simulink model "district_heating_r04"  (R2018b)
settings: Solver=ode45  StartTime=0.0  StopTime=24*3600  RelTol=1e-3
undefined symbols (not defined in the file): DPConstant, DPLinear, DPQuadratic, FluidMix, ID, MassFlow, path_carnot, Temperature
libraries: carnot x12, Pipe_BiFlow x2
settings Model: Creator=drhf  LastModifiedBy=drhf
settings SolverCC: AlgebraicLoopSolver=LineSearch

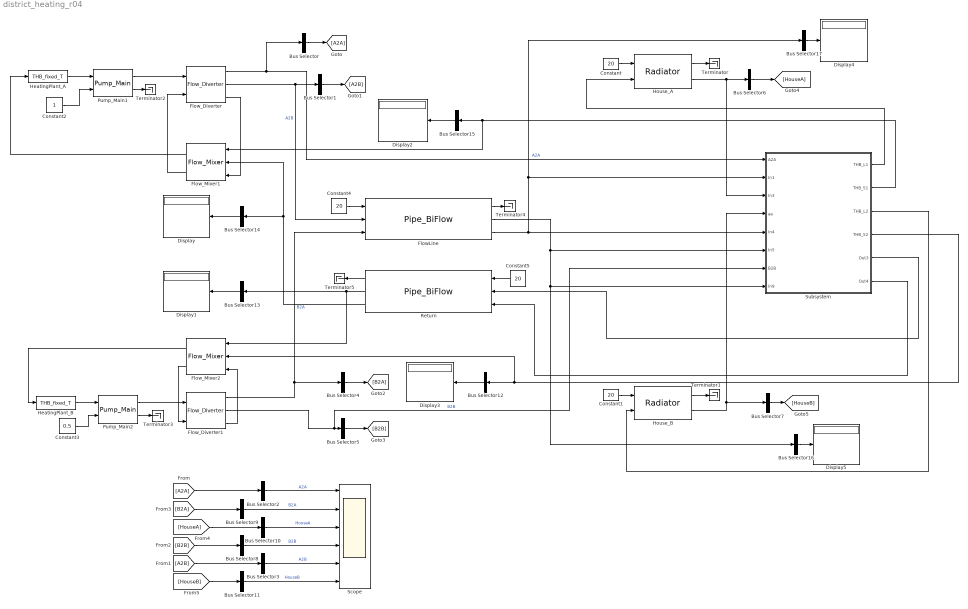
== system district_heating_r04 ==
  Bus Selector{,1,4..7} (6 alike) : BusSelector  OutputSignals=Temperature,MassFlow  OutputAsBus=on
  Bus Selector{2..3,8..11} (6 alike) : BusSelector  OutputSignals=MassFlow  OutputAsBus=on
  Bus Selector{12..17} (6 alike) : BusSelector  OutputSignals=MassFlow,DPConstant,DPLinear,DPQuadratic  OutputAsBus=on
  Constant{,1,4..5} (4 alike) : Constant  Value=20
  Constant2 : Constant
  Constant3 : Constant  Value=0.5
  Display{,1..5} (6 alike) : Display
  FlowLine : Pipe_BiFlow/Pipe_BiFlow  t0=20  hgt=254.6479  stgtype=1  tini=[20 20 20 20 20 20 20 20 20 20]  mpts=[1 2 3 4 5 6 7 8 9 10]  PathName=fullfile(path_carnot('libsl'),'Storage','Thermal','Storage_Type_1','parameter_set')  FileName='<user defined>'  userPath=off  userParam=on  uwall=1  ubot=1  utop=1  axcond=1  volume=2  dia=0.1  standing=standing cylinder  nodes=10  mpoints=10  pipe1inlet=1  pipe1outlet=0  pipe1dia=0.1  pipe2inlet=0  pipe2outlet=1  pipe2dia=0.1
  Flow_Diverter : carnot/Hydraulics/Flow_Diverter
      settings: SourceProductName=Carnot
  Flow_Diverter1 : carnot/Hydraulics/Flow_Diverter
      settings: SourceProductName=Carnot
  Flow_Mixer1 : carnot/Hydraulics/Flow_Mixer
      settings: SourceProductName=Carnot
  Flow_Mixer2 : carnot/Hydraulics/Flow_Mixer
      settings: SourceProductName=Carnot
  HeatingPlant_A : carnot/Source/Simple/THB_fixed_T  t=70
      settings: SourceProductName=Carnot
  HeatingPlant_B : carnot/Source/Simple/THB_fixed_T  t=60
      settings: SourceProductName=Carnot
  House_A : carnot/Source/Heat_Exchanger/Radiator  pnom=500  dtnom=49.83  expo=1.3  mcap=5*4182  tini=20  lin=10  qua=10
      settings: SourceProductName=Carnot
  House_B : carnot/Source/Heat_Exchanger/Radiator  pnom=500  dtnom=49.83  expo=1.3  mcap=5*4182  tini=20  lin=10  qua=10
      settings: SourceProductName=Carnot
  Pump_Main1 : carnot/Hydraulics/Pump_Main  Tini=20  p0=3e5  IDpreset=pressure drop  fluid=Water  mix=0  mix2=0  mix3=0  t1=5  PathName=fullfile(path_carnot('libsl'), 'Hydraulics', 'Pump_Main', 'parameter_set')  FileName='Pump8m.mat'  userPath=off  userParam=off  a0=80000  a1=-32000  a2=0  dia=0.025  UA=1  mcp=4182  e0=100  e1=36  e2=-6.4
      settings: SourceProductName=Carnot
  Pump_Main2 : carnot/Hydraulics/Pump_Main  Tini=20  p0=3e5  IDpreset=pressure drop  fluid=Water  mix=0  mix2=0  mix3=0  t1=1  PathName=fullfile(path_carnot('libsl'), 'Hydraulics', 'Pump_Main', 'parameter_set')  FileName='Pump8m.mat'  userPath=off  userParam=off  a0=80000  a1=-32000  a2=0  dia=0.025  UA=1  mcp=4182  e0=100  e1=36  e2=-6.4
      settings: SourceProductName=Carnot
  Return : Pipe_BiFlow/Pipe_BiFlow  t0=20  hgt=254.6479  stgtype=1  tini=[20 20 20 20 20 20 20 20 20 20]  mpts=[1 2 3 4 5 6 7 8 9 10]  PathName=fullfile(path_carnot('libsl'),'Storage','Thermal','Storage_Type_1','parameter_set')  FileName='<user defined>'  userPath=off  userParam=on  uwall=1  ubot=1  utop=1  axcond=1  volume=2  dia=0.1  standing=standing cylinder  nodes=10  mpoints=10  pipe1inlet=1  pipe1outlet=0  pipe1dia=0.1  pipe2inlet=0  pipe2outlet=1  pipe2dia=0.1
  Scope : Scope  NumInputPorts=6
  Subsystem : Subsystem
  Terminator{,1..5} (6 alike) : Terminator
  wires:
  Constant/1 -> House_A/1
  House_A/1 -> Terminator/1
  HeatingPlant_B/1 -> Pump_Main2/1
  HeatingPlant_A/1 -> Pump_Main1/1
  House_B/1 -> Terminator1/1
  Constant1/1 -> House_B/1
  Pump_Main1/2 -> Terminator2/1
  Pump_Main2/2 -> Terminator3/1
  Constant2/1 -> Pump_Main1/2
  Constant3/1 -> Pump_Main2/2
  Constant4/1 -> FlowLine/1
  Pump_Main1/1 -> Flow_Diverter/1
  Pump_Main2/1 -> Flow_Diverter1/1
  FlowLine/1 -> Terminator4/1
  Constant5/1 -> Return/1
  Flow_Diverter/1 -> Bus Selector/1, Subsystem/1(A2A)  "A2A"
  Flow_Diverter1/2 -> Subsystem/7(B2B), Bus Selector5/1  "B2B"
  Return/1 -> Terminator5/1
  Flow_Diverter1/3 -> Flow_Mixer2/3
  Flow_Mixer2/2 -> Flow_Diverter1/2
  Flow_Mixer1/2 -> Flow_Diverter/2
  Flow_Diverter/3 -> Flow_Mixer1/3
  Bus Selector/1 -> [A2A]
  Bus Selector1/1 -> [A2B]
  Flow_Diverter/2 -> Bus Selector1/1, FlowLine/2  "A2B"
  [A2A] -> Bus Selector2/1
  Bus Selector2/1 -> Scope/1  "A2A"
  [A2B] -> Bus Selector3/1
  Bus Selector3/1 -> Scope/5  "A2B"
  Flow_Diverter1/1 -> FlowLine/3, Bus Selector4/1  "B2A"
  Bus Selector4/1 -> [B2A]
  Bus Selector5/1 -> [B2B]
  Bus Selector6/1 -> [HouseA]
  Bus Selector7/1 -> [HouseB]
  [B2B] -> Bus Selector8/1
  [B2A] -> Bus Selector9/1
  [HouseA] -> Bus Selector10/1
  [HouseB] -> Bus Selector11/1
  Bus Selector8/1 -> Scope/4  "B2B"
  Bus Selector9/1 -> Scope/2  "B2A"
  Bus Selector10/1 -> Scope/3  "HouseA"
  Bus Selector11/1 -> Scope/6  "HouseB"
  Flow_Mixer1/1 -> HeatingPlant_A/1
  Flow_Mixer2/1 -> HeatingPlant_B/1
  Return/3 -> Flow_Mixer1/2, Bus Selector14/1
  Return/2 -> Flow_Mixer2/1, Bus Selector13/1
  Bus Selector14/1 -> Display/1
  Bus Selector13/1 -> Display1/1
  Bus Selector15/1 -> Display2/1
  Bus Selector12/1 -> Display3/1
  Bus Selector16/1 -> Display5/1
  Bus Selector17/1 -> Display4/1
  House_A/2 -> Subsystem/3(In3), Bus Selector6/1
  House_B/2 -> Subsystem/4(aa), Bus Selector7/1
  FlowLine/3 -> Bus Selector17/1, Subsystem/2(In1), Subsystem/5(In4)
  FlowLine/2 -> Bus Selector16/1, Subsystem/8(In9), Subsystem/6(In5)
  Subsystem/4(THB_S2) -> Flow_Mixer2/2, Bus Selector12/1
  Subsystem/2(THB_S1) -> Flow_Mixer1/1, Bus Selector15/1
  Subsystem/1(THB_L1) -> House_A/2
  Subsystem/5(Out3) -> Return/2
  Subsystem/6(Out4) -> Return/3
  Subsystem/3(THB_L2) -> House_B/2

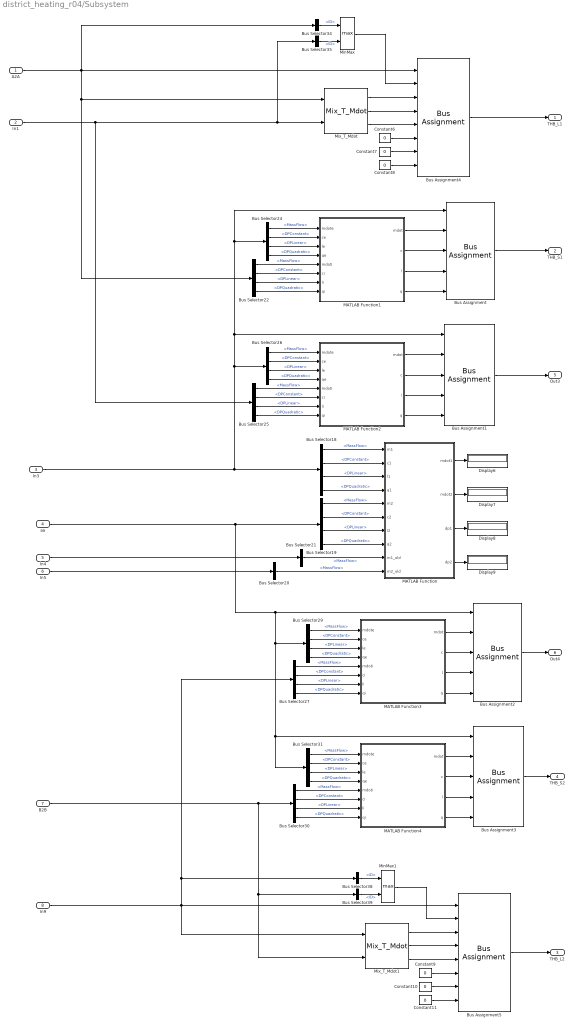
== system district_heating_r04/Subsystem ==
  A2A : Inport
  In1 : Inport  Port=2
  In3 : Inport  Port=3
  aa : Inport  Port=4
  In4 : Inport  Port=5
  In5 : Inport  Port=6
  B2B : Inport  Port=7
  In9 : Inport  Port=8
  Bus Assignment{,1..3} (4 alike) : BusAssignment  AssignedSignals=MassFlow,DPConstant,DPLinear,DPQuadratic
  Bus Assignment4 : BusAssignment  AssignedSignals=ID,Temperature,MassFlow,FluidMix,DPConstant,DPLinear,DPQuadratic
  Bus Assignment5 : BusAssignment  AssignedSignals=ID,Temperature,MassFlow,FluidMix,DPConstant,DPLinear,DPQuadratic
  Bus Selector{18..19,22,24..27,29..31} (10 alike) : BusSelector  OutputSignals=MassFlow,DPConstant,DPLinear,DPQuadratic
  Bus Selector20 : BusSelector  OutputSignals=MassFlow
  Bus Selector21 : BusSelector  OutputSignals=MassFlow
  Bus Selector{34..35,38..39} (4 alike) : BusSelector  OutputSignals=ID
  Constant{6..11} (6 alike) : Constant  Value=0
  Display{6..9} (4 alike) : Display
  MATLAB Function : MATLAB Function  TreatAsAtomicUnit=on
  MATLAB Function1 : MATLAB Function  TreatAsAtomicUnit=on
  MATLAB Function2 : MATLAB Function  TreatAsAtomicUnit=on
  MATLAB Function3 : MATLAB Function  TreatAsAtomicUnit=on
  MATLAB Function4 : MATLAB Function  TreatAsAtomicUnit=on
  MinMax : MinMax  Function=max  Inputs=2
  MinMax1 : MinMax  Function=max  Inputs=2
  Mix_T_Mdot : carnot/Basic/Hydraulics/Mix_T_Mdot  mixcalc=Tmix = (mdot1*T1 + mdot2*T2)/(mdot1+mdot2)
      settings: SourceProductName=Carnot
  Mix_T_Mdot1 : carnot/Basic/Hydraulics/Mix_T_Mdot  mixcalc=Tmix = (mdot1*T1 + mdot2*T2)/(mdot1+mdot2)
      settings: SourceProductName=Carnot
  THB_L1 : Outport
  THB_S1 : Outport  Port=2
  THB_L2 : Outport  Port=3
  THB_S2 : Outport  Port=4
  Out3 : Outport  Port=5
  Out4 : Outport  Port=6
  wires:
  MATLAB Function/1(mdot1) -> Display6/1
  Bus Selector19/3 -> MATLAB Function/7(l2)  "<DPLinear>"
  Constant11/1 -> Bus Assignment5/8
  In3/1 -> Bus Assignment/1, Bus Selector24/1, Bus Assignment1/1, Bus Selector26/1, Bus Selector18/1
  Bus Selector31/4 -> MATLAB Function4/4(qe)  "<DPQuadratic>"
  Mix_T_Mdot/2 -> Bus Assignment4/4
  Bus Selector25/2 -> MATLAB Function2/6(ci)  "<DPConstant>"
  MinMax/1 -> Bus Assignment4/2
  Mix_T_Mdot/1 -> Bus Assignment4/3
  Bus Selector18/2 -> MATLAB Function/2(c1)  "<DPConstant>"
  Bus Selector30/2 -> MATLAB Function4/6(ci)  "<DPConstant>"
  MATLAB Function4/2(c) -> Bus Assignment3/3
  Constant9/1 -> Bus Assignment5/6
  MATLAB Function3/4(q) -> Bus Assignment2/5
  In9/1 -> Bus Selector27/1, Bus Selector38/1, Mix_T_Mdot1/1, Bus Assignment5/1
  Bus Selector29/4 -> MATLAB Function3/4(qe)  "<DPQuadratic>"
  MATLAB Function1/1(mdot) -> Bus Assignment/2
  Constant6/1 -> Bus Assignment4/6
  Bus Selector30/4 -> MATLAB Function4/8(qi)  "<DPQuadratic>"
  Bus Selector22/2 -> MATLAB Function1/6(ci)  "<DPConstant>"
  Bus Selector27/3 -> MATLAB Function3/7(li)  "<DPLinear>"
  Constant8/1 -> Bus Assignment4/8
  Bus Selector29/2 -> MATLAB Function3/2(ce)  "<DPConstant>"
  MATLAB Function2/3(l) -> Bus Assignment1/4
  Bus Selector18/1 -> MATLAB Function/1(m1)  "<MassFlow>"
  aa/1 -> Bus Selector31/1, Bus Assignment3/1, Bus Selector29/1, Bus Assignment2/1, Bus Selector19/1
  Bus Selector35/1 -> MinMax/2  "<ID>"
  Bus Selector26/2 -> MATLAB Function2/2(ce)  "<DPConstant>"
  Bus Assignment5/1 -> THB_L2/1
  Bus Selector29/3 -> MATLAB Function3/3(le)  "<DPLinear>"
  Bus Selector27/1 -> MATLAB Function3/5(mdoti)  "<MassFlow>"
  Constant7/1 -> Bus Assignment4/7
  Bus Selector24/1 -> MATLAB Function1/1(mdote)  "<MassFlow>"
  Mix_T_Mdot/3 -> Bus Assignment4/5
  Bus Selector24/4 -> MATLAB Function1/4(qe)  "<DPQuadratic>"
  Bus Selector18/4 -> MATLAB Function/4(q1)  "<DPQuadratic>"
  Bus Selector18/3 -> MATLAB Function/3(l1)  "<DPLinear>"
  Bus Selector19/2 -> MATLAB Function/6(c2)  "<DPConstant>"
  A2A/1 -> Bus Selector34/1, Bus Selector22/1, Mix_T_Mdot/1, Bus Assignment4/1
  Bus Selector20/1 -> MATLAB Function/10(m2_old)  "<MassFlow>"
  MATLAB Function4/1(mdot) -> Bus Assignment3/2
  B2B/1 -> Mix_T_Mdot1/2, Bus Selector39/1, Bus Selector30/1
  MATLAB Function4/3(l) -> Bus Assignment3/4
  Bus Selector27/2 -> MATLAB Function3/6(ci)  "<DPConstant>"
  Bus Selector25/1 -> MATLAB Function2/5(mdoti)  "<MassFlow>"
  Bus Selector31/2 -> MATLAB Function4/2(ce)  "<DPConstant>"
  MATLAB Function2/4(q) -> Bus Assignment1/5
  MATLAB Function3/2(c) -> Bus Assignment2/3
  Bus Selector38/1 -> MinMax1/1  "<ID>"
  Bus Selector26/1 -> MATLAB Function2/1(mdote)  "<MassFlow>"
  Bus Selector19/1 -> MATLAB Function/5(m2)  "<MassFlow>"
  Bus Selector19/4 -> MATLAB Function/8(q2)  "<DPQuadratic>"
  Bus Selector31/1 -> MATLAB Function4/1(mdote)  "<MassFlow>"
  Bus Selector25/3 -> MATLAB Function2/7(li)  "<DPLinear>"
  MinMax1/1 -> Bus Assignment5/2
  MATLAB Function/4(dp2) -> Display9/1
  Bus Selector22/3 -> MATLAB Function1/7(li)  "<DPLinear>"
  Bus Selector30/1 -> MATLAB Function4/5(mdoti)  "<MassFlow>"
  Bus Selector29/1 -> MATLAB Function3/1(mdote)  "<MassFlow>"
  MATLAB Function3/1(mdot) -> Bus Assignment2/2
  In5/1 -> Bus Selector20/1
  MATLAB Function4/4(q) -> Bus Assignment3/5
  MATLAB Function/2(mdot2) -> Display7/1
  Bus Selector34/1 -> MinMax/1  "<ID>"
  Bus Selector24/2 -> MATLAB Function1/2(ce)  "<DPConstant>"
  Constant10/1 -> Bus Assignment5/7
  Bus Selector24/3 -> MATLAB Function1/3(le)  "<DPLinear>"
  MATLAB Function1/2(c) -> Bus Assignment/3
  Bus Selector22/1 -> MATLAB Function1/5(mdoti)  "<MassFlow>"
  Bus Selector22/4 -> MATLAB Function1/8(qi)  "<DPQuadratic>"
  Bus Selector25/4 -> MATLAB Function2/8(qi)  "<DPQuadratic>"
  MATLAB Function2/2(c) -> Bus Assignment1/3
  Bus Selector30/3 -> MATLAB Function4/7(li)  "<DPLinear>"
  MATLAB Function3/3(l) -> Bus Assignment2/4
  Bus Selector27/4 -> MATLAB Function3/8(qi)  "<DPQuadratic>"
  Mix_T_Mdot1/2 -> Bus Assignment5/4
  Bus Selector31/3 -> MATLAB Function4/3(le)  "<DPLinear>"
  In1/1 -> Bus Selector25/1, Bus Selector35/1, Mix_T_Mdot/2
  MATLAB Function1/3(l) -> Bus Assignment/4
  Bus Selector21/1 -> MATLAB Function/9(m1_old)  "<MassFlow>"
  Bus Selector26/4 -> MATLAB Function2/4(qe)  "<DPQuadratic>"
  Bus Selector26/3 -> MATLAB Function2/3(le)  "<DPLinear>"
  MATLAB Function1/4(q) -> Bus Assignment/5
  MATLAB Function2/1(mdot) -> Bus Assignment1/2
  MATLAB Function/3(dp1) -> Display8/1
  Mix_T_Mdot1/1 -> Bus Assignment5/3
  Mix_T_Mdot1/3 -> Bus Assignment5/5
  Bus Selector39/1 -> MinMax1/2  "<ID>"
  In4/1 -> Bus Selector21/1
  Bus Assignment2/1 -> Out4/1
  Bus Assignment1/1 -> Out3/1
  Bus Assignment3/1 -> THB_S2/1
  Bus Assignment/1 -> THB_S1/1
  Bus Assignment4/1 -> THB_L1/1

== matlab function district_heating_r04/Subsystem/MATLAB Function3 ==
  data: mdot output; mdote input; c output; ce input; le input; qe input; l output; q output; mdoti input; ci input; li input; qi input
function [mdot, c, l, q] = distributorBar_recalc_clq(mdote, ce, le, qe, mdoti, ci, li, qi)

% Basic equations:
% pressure drop dp = c + l*mdot + q*mdot^2

noMassflow = sqrt(eps(100));  % assume no massflow below this limit

% Massflow mdoti in the branch is given via info inport .
mdot = mdoti; % massflow is flow from info input

% Entering flow mdote and its coeffs (ce, le, qe) must be replaced by
% mdoti  with coeffs c, l, q fullfilling the condition that
% calulated pressure drop in entering pipe is maintained
%  dp = ce + le*mdote + qe*mdote^2 =  c + l*mdoti + q*mdoti^2 
% for all massflows mdote and mdoti
% -> c = ce
% -> l = le*mdote/mdoti
% -> q = qe*mdote^2/mdoti^2
c = ce;
if mdoti < noMassflow
    l = le;
    q = qe;
else
    v = mdote/mdoti;
    l = le*v;
    q = qe*v^2;
end

% additional pressure drop from the info inport must be added
c = c + ci;
l = l + li;
q = q + qi;

== matlab function district_heating_r04/Subsystem/MATLAB Function4 ==
  data: mdot output; mdote input; c output; ce input; le input; qe input; l output; q output; mdoti input; ci input; li input; qi input
function [mdot, c, l, q] = distributorBar_recalc_clq(mdote, ce, le, qe, mdoti, ci, li, qi)

% Basic equations:
% pressure drop dp = c + l*mdot + q*mdot^2

noMassflow = sqrt(eps(100));  % assume no massflow below this limit

% Massflow mdoti in the branch is given via info inport .
mdot = mdoti; % massflow is flow from info input

% Entering flow mdote and its coeffs (ce, le, qe) must be replaced by
% mdoti  with coeffs c, l, q fullfilling the condition that
% calulated pressure drop in entering pipe is maintained
%  dp = ce + le*mdote + qe*mdote^2 =  c + l*mdoti + q*mdoti^2 
% for all massflows mdote and mdoti
% -> c = ce
% -> l = le*mdote/mdoti
% -> q = qe*mdote^2/mdoti^2
c = ce;
if mdoti < noMassflow
    l = le;
    q = qe;
else
    v = mdote/mdoti;
    l = le*v;
    q = qe*v^2;
end

% additional pressure drop from the info inport must be added
c = c + ci;
l = l + li;
q = q + qi;

== matlab function district_heating_r04/Subsystem/MATLAB Function ==
  data: m1 input; mdot1 output; c1 input; l1 input; q1 input; mdot2 output; m2 input; c2 input; l2 input; q2 input; m1_old input; m2_old input; dp1 output; dp2 output
function [mdot1, mdot2, dp1, dp2] = compare_dp(m1, c1, l1, q1, m2, c2, l2, q2, m1_old, m2_old)
% compare pressure drop and decide which one is dominant
dp1 = c1 + l1*m1 + q1*m1^2;
dp2 = c2 + l2*m2 + q2*m2^2;
no_dp = eps(1000);   % no pressure drop for 1000  x calculation precision

if dp1 > dp2 + no_dp
    mdot1 = 0;
    mdot2 = m2_old;
elseif dp2 > dp1 + no_dp
    mdot1 = m1_old;
    mdot2 = 0;
else
    mdot1 = 0;
    mdot2 = 0;
end

== matlab function district_heating_r04/Subsystem/MATLAB Function1 ==
  data: mdot output; mdote input; c output; ce input; le input; qe input; l output; q output; mdoti input; ci input; li input; qi input
function [mdot, c, l, q] = distributorBar_recalc_clq(mdote, ce, le, qe, mdoti, ci, li, qi)

% Basic equations:
% pressure drop dp = c + l*mdot + q*mdot^2

noMassflow = sqrt(eps(100));  % assume no massflow below this limit

% Massflow mdoti in the branch is given via info inport .
mdot = mdoti; % massflow is flow from info input

% Entering flow mdote and its coeffs (ce, le, qe) must be replaced by
% mdoti  with coeffs c, l, q fullfilling the condition that
% calulated pressure drop in entering pipe is maintained
%  dp = ce + le*mdote + qe*mdote^2 =  c + l*mdoti + q*mdoti^2 
% for all massflows mdote and mdoti
% -> c = ce
% -> l = le*mdote/mdoti
% -> q = qe*mdote^2/mdoti^2
c = ce;
if mdoti < noMassflow
    l = le;
    q = qe;
else
    v = mdote/mdoti;
    l = le*v;
    q = qe*v^2;
end

% additional pressure drop from the info inport must be added
c = c + ci;
l = l + li;
q = q + qi;

== matlab function district_heating_r04/Subsystem/MATLAB Function2 ==
  data: mdot output; mdote input; c output; ce input; le input; qe input; l output; q output; mdoti input; ci input; li input; qi input
function [mdot, c, l, q] = distributorBar_recalc_clq(mdote, ce, le, qe, mdoti, ci, li, qi)

% Basic equations:
% pressure drop dp = c + l*mdot + q*mdot^2

noMassflow = sqrt(eps(100));  % assume no massflow below this limit

% Massflow mdoti in the branch is given via info inport .
mdot = mdoti; % massflow is flow from info input

% Entering flow mdote and its coeffs (ce, le, qe) must be replaced by
% mdoti  with coeffs c, l, q fullfilling the condition that
% calulated pressure drop in entering pipe is maintained
%  dp = ce + le*mdote + qe*mdote^2 =  c + l*mdoti + q*mdoti^2 
% for all massflows mdote and mdoti
% -> c = ce
% -> l = le*mdote/mdoti
% -> q = qe*mdote^2/mdoti^2
c = ce;
if mdoti < noMassflow
    l = le;
    q = qe;
else
    v = mdote/mdoti;
    l = le*v;
    q = qe*v^2;
end

% additional pressure drop from the info inport must be added
c = c + ci;
l = l + li;
q = q + qi;
